simulink model "Explorer1632_dsPIC33EP512MU810_UART_Terminal_R2017b"  (R2017b)
settings: Solver=FixedStepDiscrete  StartTime=0.0  StopTime=inf  FixedStep=0.01  RelTol=1e-3  EnableMultiTasking=on
undefined symbols (not defined in the file): A0, D0, DiscIntNeverNeededParam, F4, F5, Max, ms, P100, P101, P16, P64, Pin, Resol, us
libraries: MCHP_Blockset x40, simulink x11
(part 1 of 2)
settings Model: ExtModeTrigDuration=1  Creator=M17129  LastModifiedBy=Lubin Kerhuel
settings OptimizationCC: DefaultParameterBehavior=Inlined  DefaultUnderspecifiedDataType=single  BooleansAsBitfields=on  PassReuseOutputArgsAs=Individual arguments
settings DebuggingCC: InheritedTsInSrcMsg=none  ParameterTunabilityLossMsg=error
settings HardwareCC: ProdBitPerInt=16  ProdBitPerPointer=32  ProdBitPerSizeT=16  ProdBitPerPtrDiffT=16  ProdLargestAtomicInteger=Integer  ProdLargestAtomicFloat=None  ProdWordSize=16  ProdHWDeviceType=Generic->Custom
settings ModelReferenceCC: ModelReferenceNumInstancesAllowed=Single
settings SFSimCC: MATLABDynamicMemAlloc=off
settings RTWCC: Description=Microchip Embedded Target PIC24 dsPIC30 dsPIC33 (real-time)  SystemTargetFile=MCHP_dsPIC_stf.tlc  TemplateMakefile=MCHP_dsPIC.tmf  GenerateReport=on  CustomInclude=./  CustomSource=code.c  IncludeHyperlinkInReport=on  LaunchReport=on  GenerateTraceInfo=on  GenerateTraceReport=on  GenerateTraceReportSl=on  GenerateTraceReportSf=on  GenerateTraceReportEml=on  GenerateWebview=on  GenerateCodeMetricsReport=on  GenerateCodeReplacementReport=on
settings CodeAppCC: ForceParamTrailComments=on  IgnoreCustomStorageClasses=off  MaxIdLength=255  OperatorAnnotations=on  SimulinkDataObjDesc=on  SFDataObjDesc=on  InsertBlockDesc=on
settings STFCustomTargetCC: TargetLibSuffix=_lib.a  MultiwordLength=256  IncludeMdlTerminateFcn=off  CombineOutputUpdateFcns=on  CombineSignalStateStructs=on  SuppressErrorStatus=on  ERTCustomFileBanners=on  SupportContinuousTime=off  RemoveResetFunc=on  MATLABClassNameForMDSCustomization=Simulink.SoftwareTarget.ERTCustomization  GRTInterface=off  SystemTargetFile=MCHP_dsPIC_stf.tlc
settings ERTTargetCC: TargetLibSuffix=_lib.a  ParMdlRefBuildCompliant=off  CompOptLevelCompliant=off  ConcurrentExecutionCompliant=off  IncludeMdlTerminateFcn=off  CombineSignalStateStructs=on  SuppressErrorStatus=on  SupportNonInlinedSFcns=on  ModelStepFunctionPrototypeControlCompliant=off  CPPClassGenCompliant=off  UseToolchainInfoCompliant=off  ExtModeStaticAllocSize=500  InlinedParameterPlacement=NonHierarchical  ERTSrcFileBannerTemplate=MCHP_dsPIC_code_template.cgt  ERTHdrFileBannerTemplate=MCHP_dsPIC_code_template.cgt  ERTDataSrcFileTemplate=MCHP_dsPIC_code_template.cgt  ERTDataHdrFileTemplate=MCHP_dsPIC_code_template.cgt  ERTCustomFileTemplate=MCHP_main.tlc  MemSecPackage=Simulink

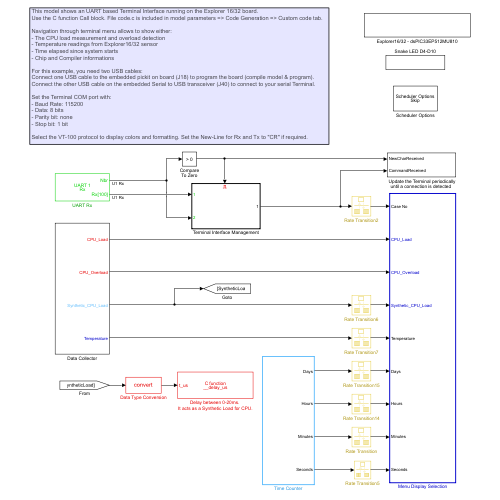
[thumbnail: Simulink's stored preview of the top-level diagram]
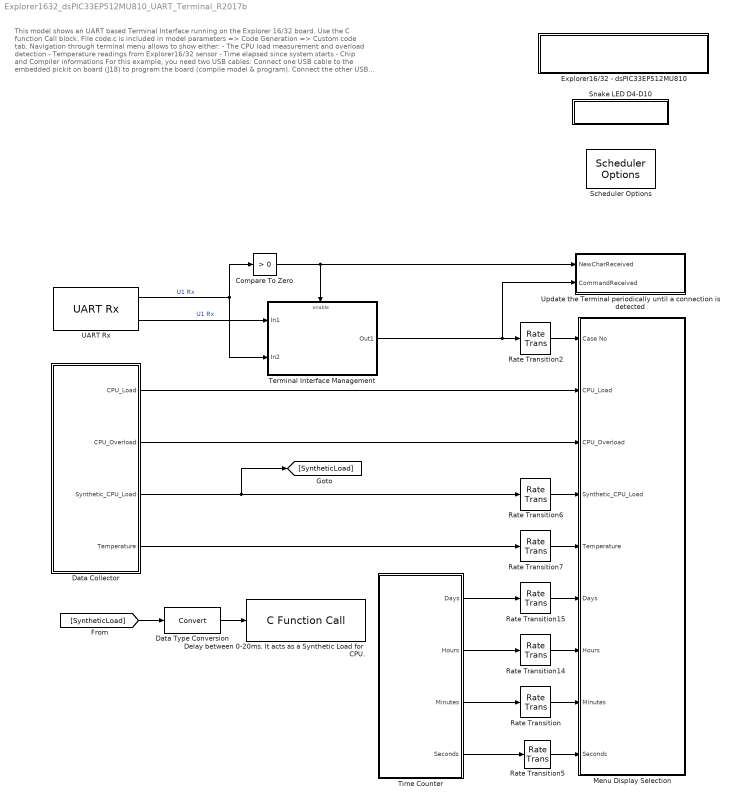
== system Explorer1632_dsPIC33EP512MU810_UART_Terminal_R2017b ==
  note: This model shows an UART based Terminal Interface running on the Explorer 16/32 board.
      | Use the C function Call block. File code.c is included in model parameters => Code Generation => Custom code tab.
      |
      | Navigation through terminal menu allows to show either:
      | - The CPU load measurement and overload detection
      | - Temperature readings from Explorer16/32 sensor
      | - Time elapsed since system starts
      | - Chip and Compiler informations
      |
      | For this example, you need two USB cables:
      | Connect one USB cable to the embedded pickit on board (J18) to program the board (compile model & program).
      | Connect the other USB cable on the embedded Serial to USB transceiver (J40) to connect to your serial Terminal.
      |
      | Set the Terminal COM port with:
      | - Baud Rate: 115200
      | - Data: 8 bits
      | - Parity bit: none
      | - Stop bit: 1 bit
      |
      | Select the VT-100 protocol to display colors and formatting. Set the New-Line for Rx and Tx to "CR" if required.
  " Update the Terminal periodically until a connection is detected " : Subsystem
  Compare To Zero : simulink/Logic and Bit Operations/Compare To Zero  relop=>  OutDataTypeStr=boolean
  Data Collector : Subsystem
  Data Type Conversion : DataTypeConversion
  Delay between 0-20ms. It acts as a Synthetic Load for CPU. : MCHP_Blockset/User Functions/C Function Call  ParseFilesChkbx=off  ListFunctions1=Custom Function  Function1=extern void __delay_us(unsigned long t_us);  AddHeaderDeclaration=off  Function1Type=when block is updated (default)  Fct1BlockIn=t_us  FctReturnBlockOut=off  DataCollected=0  ORDERING=None  SampleTime=-1  S_INPUT=0  S_INPUT_Size=0  S_OUTPUT=0  S_OUTPUT_Size=0  S_ListCustomDatatype=0  MCHP_CRC=957180  MCHP_MASTERLINK=Explorer1632_dsPIC33EP512MU810_UART_Terminal_R2017b/Explorer16//32 - dsPIC33EP512MU810/Microchip Master  PinDigitalInput=[]  PinDigitalOutput=[]  PinAnalogInput=[]
      settings: SourceProductName=MPLAB® Device Blocks for Simulink®
  Explorer16/32 - dsPIC33EP512MU810 : Subsystem
  Menu Display Selection : Subsystem  TreatAsAtomicUnit=on  SystemSampleTime=0.2
  Rate Transition{,2,5..7,14..15} (7 alike) : RateTransition  Deterministic=off  OutPortSampleTimeOpt=Inherit
  Scheduler Options : MCHP_Blockset/System Configuration/Scheduler Options  TaskOverloadBehaviour=Skip this task execution once  MCHP_MASTERLINK=UTester_33EP512MU810_CPUOverLoad/Microchip Master
      settings: SourceProductName=MPLAB® Device Blocks for Simulink®
  Snake LED D4-D10 : Subsystem
  Terminal Interface Management : Subsystem
  Time Counter : Subsystem  TreatAsAtomicUnit=on
  UART Rx : MCHP_Blockset/BUS UART/UART Rx  UART_REF=1  Flag_Out=on  Rx_Size_popup=User defined  Rx_Size=100  S_Rx_Size=100  Split=Read all received char  SplitChar=13  OutputDefault_popup=Add one trailing 0  OutputDefault=-2  ORDERING=None  SampleTime=0.01  MCHP_MASTERLINK=Explorer1632_dsPIC33EP512MU810_UART_Terminal_R2017b/Explorer16//32 - dsPIC33EP512MU810/Microchip Master  MCHP_COMPILED_INFO="CompiledSampleTime= [0.010000000000000000208   0 ];CompiledInportDataTypes=[    ];CompiledInportDataWidth=[];"
      settings: SourceProductName=MPLAB® Device Blocks for Simulink®
  wires:
  UART Rx/2 -> Terminal Interface Management/1(In1)  "U1 Rx"
  UART Rx/1 -> Terminal Interface Management/2(In2), Compare To Zero/1  "U1 Rx"
  Terminal Interface Management/1(Out1) -> Rate Transition2/1, " Update the Terminal periodically until a connection is detected "/2(CommandReceived)
  Data Collector/4(Temperature) -> Rate Transition7/1
  Time Counter/3(Minutes) -> Rate Transition/1
  Time Counter/1(Days) -> Rate Transition15/1
  Time Counter/2(Hours) -> Rate Transition14/1
  Time Counter/4(Seconds) -> Rate Transition5/1
  Rate Transition15/1 -> Menu Display Selection/6(Days)
  Rate Transition14/1 -> Menu Display Selection/7(Hours)
  Rate Transition/1 -> Menu Display Selection/8(Minutes)
  Rate Transition5/1 -> Menu Display Selection/9(Seconds)
  Compare To Zero/1 -> " Update the Terminal periodically until a connection is detected "/1(NewCharReceived), Terminal Interface Management/Enable
  Data Type Conversion/1 -> Delay between 0-20ms. It acts as a Synthetic Load for CPU./1
  Rate Transition2/1 -> Menu Display Selection/1(Case No)
  Data Collector/3(Synthetic_CPU_Load) -> [SyntheticLoad], Rate Transition6/1
  Data Collector/2(CPU_Overload) -> Menu Display Selection/3(CPU_Overload)
  Data Collector/1(CPU_Load) -> Menu Display Selection/2(CPU_Load)
  Rate Transition6/1 -> Menu Display Selection/4(Synthetic_CPU_Load)
  Rate Transition7/1 -> Menu Display Selection/5("Temperature ")
  [SyntheticLoad] -> Data Type Conversion/1

== system Explorer1632_dsPIC33EP512MU810_UART_Terminal_R2017b/ Update the Terminal periodically until a connection is detected  ==
  NewCharReceived : Inport
  CommandReceived : Inport  Port=2
  Logical Operator2 : Logic  Operator=OR  AllPortsSameDT=off  OutDataTypeStr=boolean
  Periodic update until a valid cmd is received : Subsystem
  Periodic update until first character is received : Subsystem
  Terminal Initialization : Subsystem  Priority=2
  wires:
  NewCharReceived/1 -> Periodic update until first character is received/1(NewCharReceived), Periodic update until a valid cmd is received/1(NewCharReceived)
  CommandReceived/1 -> Periodic update until a valid cmd is received/2(CommandReceived)
  Periodic update until a valid cmd is received/1(Update) -> Logical Operator2/2
  Logical Operator2/1 -> Terminal Initialization/Enable
  Periodic update until first character is received/1(Out1) -> Logical Operator2/1

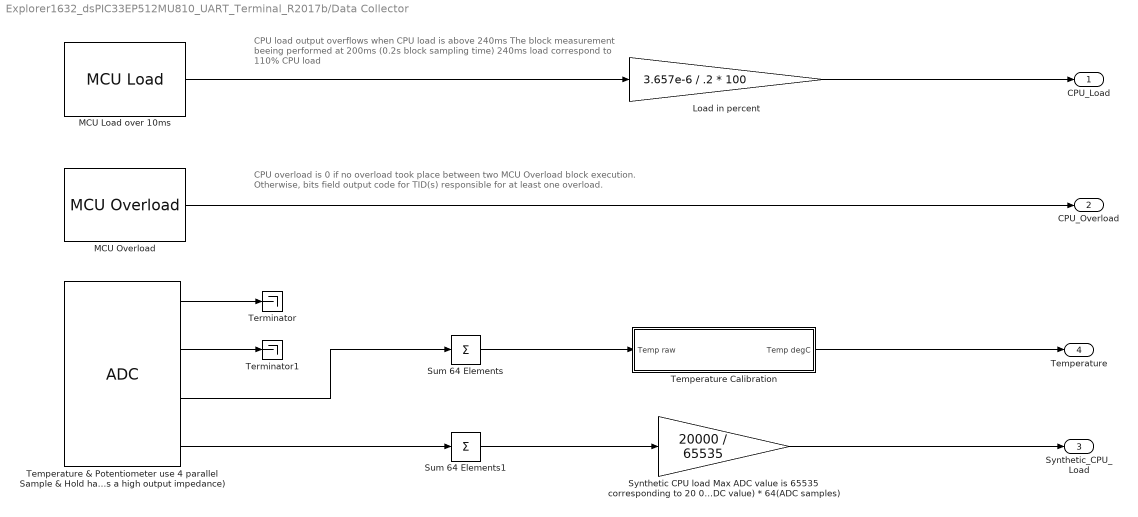
== system Explorer1632_dsPIC33EP512MU810_UART_Terminal_R2017b/Data Collector ==
  note: CPU overload is 0 if no overload took place between two MCU Overload block execution.
      | Otherwise, bits field output code for TID(s) responsible for at least one overload.
  note: CPU load output overflows when CPU load is above 240ms
      | The block measurement beeing performed at 200ms (0.2s block sampling time)
      | 240ms load correspond to 110% CPU load
  Load in percent : Gain  Gain=3.657e-6 / .2 * 100  ParamDataTypeStr=Inherit: Inherit from 'Gain'  OutMin=[0]  OutMax=[20]  OutDataTypeStr=single
  MCU Load over 10ms : MCHP_Blockset/Profiling/MCU Load  MCULoadPin=Dynamic Options  MCULoadPin_TXT=None  MCULoadMeasure=on  TIMER_Resolution=Dynamic Options  TIMER_Resolution_TXT="Resol: 3.657(us)  -  Max: 240(ms)"  MCHP_TIMER_REQUEST={MCU_Load}{MCU_Load}21:5:0:0:[]:16777216;  MCHP_TIMER_RESULT=[1 65535 ]  MCHP_MASTERLINK=Explorer1632_dsPIC33EP512MU810_UART_Terminal_R2017b/Explorer16//32 - dsPIC33EP512MU810/Microchip Master  MCHP_COMPILED_INFO="CompiledSampleTime= [0.2000000000000000111   0 ];CompiledInportDataTypes=[    ];CompiledInportDataWidth=[];"  Info="Timer 1:  Resol: 3.657142857(us)  -  Max: 239.675(ms)"  SampleTime=.2
      settings: SourceProductName=MPLAB® Device Blocks for Simulink®
  MCU Overload : MCHP_Blockset/Profiling/MCU Overload  MCUOverloadBlockOutput=on  MCUOverLoadPin=Dynamic Options  MCUOverLoadPin_TXT=None  MCHP_MASTERLINK=Explorer1632_dsPIC33EP512MU810_UART_Terminal_R2017b/Explorer16//32 - dsPIC33EP512MU810/Microchip Master  SampleTime=.2
      settings: SourceProductName=MPLAB® Device Blocks for Simulink®
  Sum 64 Elements : Sum  Inputs=+
  Sum 64 Elements1 : Sum  Inputs=+
  Synthetic CPU load Max ADC value is 65535 corresponding to 20 000us 65535(Max ADC Value) = 1024(10bit ADC value) * 64(ADC samples) : Gain  Gain=20000 / 65535  OutDataTypeStr=uint16
  Temperature & Potentiometer use 4 parallel Sample & Hold hardware (Temperature sensor has a high output impedance) : MCHP_Blockset/Analog IO/ADC  Priority=5  ADC_REF=1  Mode=10 bits (allows exact simultaneous sampling)  FORM=0000 dddd dddd dddd ==> Unsigned integer  ADC_R="< 10   kOhm"  nSAMPLECHANNELS=CH0 : CH1 : CH2 : CH3  nSAMPLECHANNELS_12bits=CH0 only  SIMULTANEOUS=Simultaneously on all Channels  ADxCSS=[0]  MUXA_CH0N=off  MUXA_CH123=Dynamic Options  MUXA_CH123_TXT=AN3 : AN4 : AN5  MUXB_CH0=AN1  MUXB_CH0N=on  MUXB_CH123=Dynamic Options  MUXB_CH123_TXT=AN0 : AN1 : AN2  SequenceRepeat=64  SequenceTiming=are stretcheded to fit exactly previous time step  SSRC_SSRCG=Dynamic Options  SSRC_SSRCG_TXT=6  Update_BlockOutput=After all trig and conversion sequence  Trig_TimeStep=with each update of the ADC block output  ADC_DMA_CHANNEL=use DMA Channel 0  SampleTime=0.01  Info=Total Time for Sample & Conversion : 0.0099968s including 5.8829e-05s (x 64) sample time. Difference with time step is : 3.2e-06s  MCHP_PORT={Analog Input 0}{AN0}15:2:B0;{Analog Input 3}{AN3}15:2:B3;{Analog Input 4}{AN4}15:2:B4;{Analog Input 5}{AN5}15:2:B5;  MCHP_MASTERLINK=Explorer1632_dsPIC33EP512MU810_UART_Terminal_R2017b/Explorer16//32 - dsPIC33EP512MU810/Microchip Master  ADC_TIMING=[0.0099968000000000001304]
      settings: SourceProductName=MPLAB® Device Blocks for Simulink®
  "Temperature Calibration " : Subsystem
  Terminator : Terminator
  Terminator1 : Terminator
  CPU_Load : Outport  VectorParamsAs1DForOutWhenUnconnected=off
  CPU_Overload : Outport  Port=2  VectorParamsAs1DForOutWhenUnconnected=off
  Synthetic_CPU_Load : Outport  Port=3  VectorParamsAs1DForOutWhenUnconnected=off
  Temperature : Outport  Port=4  VectorParamsAs1DForOutWhenUnconnected=off
  wires:
  Load in percent/1 -> CPU_Load/1
  MCU Load over 10ms/1 -> Load in percent/1
  Sum 64 Elements/1 -> "Temperature Calibration "/1(Temp raw)
  Temperature & Potentiometer use 4 parallel Sample & Hold hardware (Temperature sensor has a high output impedance)/3 -> Sum 64 Elements/1
  "Temperature Calibration "/1(Temp degC) -> Temperature/1
  Sum 64 Elements1/1 -> Synthetic CPU load Max ADC value is 65535 corresponding to 20 000us 65535(Max ADC Value) = 1024(10bit ADC value) * 64(ADC samples)/1
  Temperature & Potentiometer use 4 parallel Sample & Hold hardware (Temperature sensor has a high output impedance)/4 -> Sum 64 Elements1/1
  Synthetic CPU load Max ADC value is 65535 corresponding to 20 000us 65535(Max ADC Value) = 1024(10bit ADC value) * 64(ADC samples)/1 -> Synthetic_CPU_Load/1
  MCU Overload/1 -> CPU_Overload/1
  Temperature & Potentiometer use 4 parallel Sample & Hold hardware (Temperature sensor has a high output impedance)/1 -> Terminator/1
  Temperature & Potentiometer use 4 parallel Sample & Hold hardware (Temperature sensor has a high output impedance)/2 -> Terminator1/1

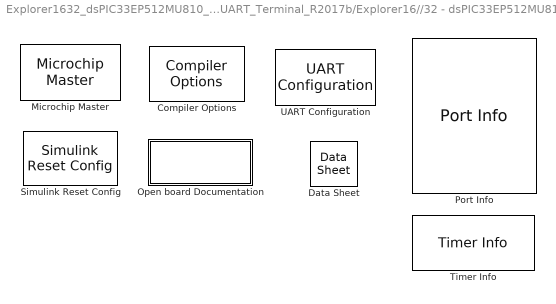
== system Explorer1632_dsPIC33EP512MU810_UART_Terminal_R2017b/Explorer16//32 - dsPIC33EP512MU810 ==
  Compiler Options : MCHP_Blockset/System Configuration/Compiler Options  Priority=1  LATEST_CMPLR=on  COMP_LIST=Dynamic Options  COMP_LIST_TXT=xc16 - v1.70  DFP_LIST=Dynamic Options  DFP_LIST_TXT=v 1.3.85  CMSIS_DSP=Dynamic Options  CMSIS_DSP_TXT=Dynamic Options  USE_64BIT_DOUBLE=off  MCHP_MULTITHREAD_COMPILATION=on  UseCustom_LinkerScript=off  MCHP_MASTERLINK=Explorer1632_dsPIC33EP512MU810_UART_Terminal_R2017b/Explorer16//32 - dsPIC33EP512MU810/Microchip Master  OPTIMIZATION_LEVEL=2  MPLAB_LINKLIB=default  MPLAB_LINKLIB1=default  CodeReplacement=Dynamic Options  CodeReplacement_TXT=None  OPTIMIZATION_FLTO=off  OPTIMIZATION_REORDER=off  UNROLL_LOOPS=off  PROCEDURAL_ABSTRACTION=off  MCODE=is less than 32768 (faster)  MCONST=in code memory  MDATA=Use only memory below address 8192 (faster)  MSCALAR=Use only memory below address 8192 (faster)  MLARGEARRAY=off  MAGGREGATE=on  HEAP_SIZE=0  OMF=elf  DEBUG_INFO=off  ProduceHexOutput=on  AssemblyListing=off  SaveTemps=off  NO_EDS_WARN=on  PRINT_STATISTICS=off
      settings: SourceProductName=MPLAB® Device Blocks for Simulink®
  Data Sheet : MCHP_Blockset/System Info/Data Sheet  DOC_Type=datasheet  DOC_MCHP_Id=33EP512MU810_datasheet  DOC_FilePath=C:\Users\M91449\AppData\Local\Temp\70616g.pdf  DOC_FileLastCheckTime="[2017              2             13             10              8         21.622]"  cpy_MCHP_Id=33EP512MU810  MCHP_MASTERLINK=Explorer1632_dsPIC33EP512MU810_UART_Terminal_R2017b/Explorer16//32 - dsPIC33EP512MU810/Microchip Master
      settings: AttributesFormatString=%<cpy_MCHP_Id>  SourceProductName=MPLAB® Device Blocks for Simulink®
  Microchip Master : MCHP_Blockset/System Configuration/Microchip Master  Priority=1  PICREF=33EP512MU810  TIMESTEP_REF="ADC  ( 0.01s + [-0.032%] ==> 0.0099968s )"  BUSYFLAG=A0 / Pin[17]  BUSYFLAG_TXT=A0 / Pin[17]  VDD_range=Dynamic Options  PWRTEN=Not used  BOREN=Disable  BODENV=2.7V  BORV=Not used  FPWRT=128ms  DSBOREN=Enable ZPBOR during Deep Sleep Mode  DSLPBOR=Not used  MCLRE=Enabled  SMCLR=MCLR pin generates a normal system Reset  PMDL1WAY=Allow only one reconfiguration  RSTPRI=Device will obtain reset instruction from Primary flash  TEMP=Not used  SOSCSRC=Not used  SOSCSEL=Not used  IOL1WAY=Allow only one reconfiguration  ALTVREF=Not used  DISUVREG=Not used  DSSWEN=Not used  LPCFG=Not used  RTCBAT=Not used  VBTBOR=Not used  WUTSEL=Not used  POWERSAVE=off  FNOSC=Primary Oscillator (XT; HS; EC)  FPR=ECIO w/ PLL 16x  FOSFPR=HS3 w/PLL 16x  FOS=Internal Fast RC  FRANGE=High Range  OSCILLATOR_SELECT=Crystal / Ceramic resonator  OSCILLATOR_SELECT_spd=Crystal / Ceramic resonator  QUARTZ=8e+06  QUARTZ_spd=8e+06  POSCGAIN=2x gain setting  POSCBOOST=Boost the kick start of the oscillator  SOSCGAIN=2x gain setting  SOSCBOOST=Boost the kick start of the oscillator  ACTIV_PLL=on  ACTIV_PLL_spd=on  MIPS_DESIRED=70e+06  MIPS_DESIRED_spd=70e+06  CPUDIV=Divide by 1  FPLLMUL=Not used  FPLLIDIV=8x Divider  POSCFREQ=Not used  POSCMD=XT Crystal Oscillator Mode  POSCMOD=Primary Oscillator Disabled  MIPS=70 * 1e6  ACLKCON=Optimized for PWM resolution & ADC conversion speed  ACLKCON_spd=Optimized for PWM resolution & ADC conversion speed  ACLKCON_Info=use FRC with auxilliary PLL, ADC Tad = 14.286(ns), PWM max resolution = 1.06(ns)  FPLLODIV=32x Divider  PLLKEN=Clock switch to PLL source will wait until the PLL lock signal is valid  FCKSM=Clock switching is enabled;Fail-safe Clock Monitor is disabled  FCKSMEN=Sw Disabled; Mon Disabled  IESO=Start up with FRC; then switch  DSWDTPS=1:2^36  FWDTEN=Disable  FWDTWINSZ=Window size is 25%  FWPSA=1:512  FWPSA0=1:128  FWPSB=1:16  WDT=Disable  WDTPOST=1:32768  WDTPRE=1:128  WDTPS=1:32768  WINDIS=Watchdog Timer in Non-Window mode  WWDTEN=Non-Window mode  DSWDTEN=Enable DSWDT during Deep Sleep Mode  DSWDTOSC=Select LPRC as DSWDT Reference clock  FPBDIV=Not used  FSOSCEN=Disable Secondary Oscillator  LPRCSEL=Not used  OSCIOFCN=Not used  OSCIOFNC=general purpose digital I/O pin  LVRCFG=Not used  PLL_96MHZ=Not used  PLL96MHZ=Not used  PLLDIV=Not used  WDTCLK=Not used  WDTCMX=Not used  WDTWIN=WDT Window is 25% of WDT period  XTCFG=24-32 MHz crystals  XTBST=Boost the kick-start  APL=Aux Flash Code protect is disabled  APLK=Aux Flash Write Protection and Code Protection is Disabled  AWRP=Auxiliary program memory is not write-protected  BSS=No Protection (other than BWRP)  BWP=Not used  BWRP=Boot Segment may be written  CP=Protection Disabled  EBS=No Boot EEPROM  ESS=No Segment Data EEPROM  GCP=General Segment Code protect is Disabled  GSS=General Segment Code protect is Disabled  GSS0=Not used  GSSK=General Segment Write Protection and Code Protection is Disabled  GWRP=General Segment may be written  PWP=Not used  RBS=No Boot RAM  RSS=No Secure RAM  SSS=No Secure Segment  SWRP=Secure segment may be written  WPCFG=Not used  WPDIS=Not used  WPEND=Not used  WPFP=Not used  ICESEL=Communicate on PGEC1/PGED1  ICS=Communicate on PGEC1 and PGED1  JTAGEN=Disable  COE=Not used  RES=Not used  DEBUG=Debugger is disabled  BACKBUG=Not used  BKBUG=Not used  ALTI2C=I2C mapped to SDA1/SCL1 pins  ALTI2C1=SDA1/SCK1 pins are selected as the I/O pins for I2C1  ALTI2C2=SDA2/SCK2 pins are selected as the I/O pins for I2C2  ALTI2C3=I2C3 mapped to SDA3/SCL3 pins  ALTQIO=QEA1; QEB1; INDX1 are selected as inputs to QEI1  ALTSS1=SS1A is selected as the I/O pin for SPI1  CMPPOL0=Hysteresis is applied to falling edge  CMPPOL1=Hysteresis is applied to falling edge  FCANIO=Not used  FETHIO=Default Ethernet I/O  FMIIEN=MII Enabled  FSRSSEL=Not used  FUSBIDIO=Controlled by the USB Module  FVBUSONIO=Not used  HPOL=Active High  HYST0=45 mV Hysteresis  HYST1=45 mV Hysteresis  I2C1SEL=Not used  LPOL=Active High  PWMPIN=Control with PORT/TRIS regs  RTCOSC=Not used  UPLLEN=USB PLL Disabled  UPLLIDIV=Not used  ATMOD8=Not used  ALTPMP=Not used  I2C2SEL=Not used  ALTADREF=Not used  ALTCVREF=Not used  PWMLOCK=PWM registers may be written without key sequence  INT_PRIORITY_DMA=0  MCHP_TIMER_RESULT=[ ]  MCHP_PORT={Busy Flag}{Busy}0:1:A0;  MCHP_PLLRegisters="[5    243  16385     -1     -1]"  MCHPVAR=MCHP.fcy.MIPS=70000000;MCHP.fcy.SYSCLK=70000000;MCHP.fcy.ADC=70000000;MCHP.fcy.Comparator=70000000;MCHP.fcy.I2C=70000000;MCHP.fcy.SPI=70000000;MCHP.fcy.UART=70000000;MCHP.fcy.Timers=70000000;MCHP.fcy.OC=70000000;MCHP.fcy.IC=70000000;MCHP.fcy.Ports=70000000;MCHP.fcy.QEI=70000000;MCHP.PowerSave=0;MCHP.TimeStepFactor=0.99968;MCHP.TimeStep_Timer=-1;MCHP.NTIMERS=9;MCHP.id.name='33EP512MU810';MCHP.id.N=reshape([33 512 810],1,3);MCHP.id.L=reshape({ 'EP','MU',''},1,3);MCHP.id.Arch=3;MCHP.periph.PPS.reg_RPINRx=reshape([-1 1 1 1 1 -1 1 1 1 1 1 1 1 1 1 1 1 1 1 1 1 1 -1 -1 1 1 1 1 1 1 1 1 1 1 1 1 1 1 1 1 1 1 1 -1 -1 -1 1 -1 -1 -1 -1 -1 1 1 1 1 1 1 1 1 1 -1 1 1 1 -1 1 1 1 1 1 1 1 1 -1 1 1 1 1 1 1 1 1 -1 1 1 1],1,87);MCHP.PPS.dsPIC.RP=reshape([-1 -1 -1 -1 -1 -1 -1 -1 -1 -1 -1 -1 -1 -1 -1 -1 -1 -1 -1 -1 -1 -1 -1 -1 -1 -1 -1 -1 -1 -1 -1 -1 -1 -1 -1 -1 -1 -1 -1 -1 -1 -1 -1 -1 -1 -1 -1 -1 -1 -1 -1 -1 -1 -1 -1 -1 -1 -1 -1 -1 -1 -1 -1 -1 48 49 50 51 52 53 54 55 -1 -1 -1 -1 -1 -1 -1 63 64 -1 66 -1 68 69 -1 71 -1 -1 -1 -1 -1 -1 -1 -1 80 81 82 83 84 85 -1 -1 88 -1 -1 -1 92 93 -1 -1 96 97 -1 -1 -1 -1 102 -1 104 -1 -1 -1 -1 109 110 111],1,128);MCHP.PPS.dsPIC.RPI=reshape([-1 -1 -1 -1 -1 -1 -1 -1 -1 -1 -1 -1 -1 -1 -1 -1 0 1 2 3 4 5 6 7 -1 -1 -1 -1 -1 -1 14 15 16 17 18 19 20 21 22 23 24 25 26 27 28 29 30 31 -1 33 34 35 36 -1 -1 -1 -1 -1 -1 -1 44 45 46 -1 -1 -1 -1 -1 -1 -1 -1 -1 56 57 58 59 60 61 62 -1 -1 65 -1 67 -1 -1 70 -1 72 73 -1 -1 -1 -1 -1 -1 -1 -1 -1 -1 -1 -1 -1 -1 -1 -1 -1 -1 -1 -1 -1 -1 -1 -1 -1 -1 -1 -1 -1 103 -1 105 -1 -1 108],1,125);MCHP.PPS.dsPIC.RPINR_list=reshape({ '1','INT1','INT2','INT3','INT4','T1CK','T2CK','T3CK','T4CK','T5CK','T6CK','T7CK','T8CK','T9CK','IC1','IC2','IC3','IC4','IC5','IC6','IC7','IC8','OCFA','OCFB','FLT1','FLT2','FLT3','FLT4','QEIA1','QEIB1','QEINDX1','QEIHOM1','QEIA2','QEIB2','QEINDX2','QEIHOM2','U1RX','U1CTS','U2RX','U2CTS','SDI1','SCK1_in','SS1_in','44','SDI2','SCK2_in','SS2_in','48','CSDIR','CSCK','COFS','52','C1RX','C2RX','U3RX','U3CTS','U4RX','U4CTS','SDI3','SCK3_in','SS3_in','62','SDI4','SCK4_in','SS4_in','66','IC9','IC10','IC11','IC12','IC13','IC14','IC15','IC16','OCFC','SYNCI1','SYNCI2','DTCMP1','DTCMP2','DTCMP3','DTCMP4','DTCMP5','DTCMP6','DTCMP7','FLT5','FLT6','FLT7','FLT8','89','SENT1','SENT2','92'},1,92);MCHP.PPS.dsPIC.RPOR_list=reshape({ '1','U1TX','U1RTS','U2TX','U2RTS','SDO1','SCK1_out','SS1_out','SDO2','SCK2_out','SS2_out','CSDO','CSCK','COFS','C1TX','C2TX','OC1','OC2','OC3','OC4','OC5','OC6','OC7','OC8','C1OUT','C2OUT','C3OUT','U3TX','U3RTS','U4TX','U4RTS','SDO3','SCK3_out','SS3_out','SDO4','SCK4_out','SS4_out','OC9','OC10','OC11','OC12','OC13','OC14','OC15','OC16','SYNCO1','SYNCO2','QEI1CCMP','QEI2CCMP','REFCLK','C4OUT','C5OUT','52','53','54','55','56','SENT1','SENT2'},1,59);MCHP.PPS.map_RPnR_RPORx=reshape([64 65 66 67 68 69 70 71 79 80 82 84 85 87 96 97 98 99 100 101 -1 -1 104 108 109 112 113 118 120 125 126 127],1,32);MCHP.Rx=reshape([17 25 -1 72 93 87 90 -1 -1 -1 -1 38 24 6 76 94 88 89 -1 -1 -1 -1 58 23 7 77 98 52 57 -1 -1 -1 -1 59 22 8 78 99 51 56 -1 -1 -1 -1 60 21 9 81 100 49 -1 -1 -1 -1 -1 61 20 -1 82 3 50 -1 -1 -1 -1 -1 91 26 -1 83 4 -1 10 -1 -1 -1 -1 92 27 -1 84 5 -1 11 -1 -1 -1 -1 -1 32 -1 68 18 53 12 -1 -1 -1 -1 28 33 -1 69 19 -1 14 -1 -1 -1 -1 29 34 -1 70 -1 -1 -1 -1 -1 -1 -1 -1 35 -1 71 -1 -1 -1 -1 -1 -1 -1 -1 41 63 79 -1 40 96 -1 -1 -1 -1 -1 42 73 80 -1 39 97 -1 -1 -1 -1 66 43 74 47 -1 -1 95 -1 -1 -1 -1 67 44 64 48 -1 -1 1 -1 -1 -1 -1],11,16);MCHP.ADC.ANtype=reshape([3 1],1,2);MCHP.ADC.ADCONx=reshape([47103 59391 40959 263 0 0],1,6);MCHP.ADC.ADCHS_0=reshape([40863 1799],1,2);MCHP.ADC.Flags=reshape([1 0],1,2);MCHP.ADC.Buffer=reshape([16 16],1,2);MCHP.ADC.port=reshape([16 17 18 19 20 21 22 23 24 25 26 27 28 29 30 31 33 34 35 36 72 73 6 7 64 65 66 67 68 69 70 71 -1 -1 -1 -1 -1 -1 -1 -1 -1 -1 -1 -1 -1 -1 -1 -1 -1 -1 -1 -1 -1 -1 -1 -1 -1],1,57);MCHP.ADC.port_ALT=reshape([-1 -1 -1 -1],1,4);MCHP.ADC.port_VrefP=10;MCHP.ADC.port_VrefM=9;MCHP.ADC.port_AVdd=-1;MCHP.ADC.port_AVss=-1;MCHP.ADC.ADCDATA=reshape([0 0 0 0 0 0 0 0 0 0 0 0 0 0 0 0 0 0 0 0 0 0 0 0 0 0 0 0 0 0 0 0 0 0 0 0 0 0 0 0 0 0 0 0 0 0 0 0 0 0 0 0 0 0 0 0 0],1,57);MCHP.ADC.HS_SAR.TRGSRC=reshape([0 0 0 0 0 0 0 0 0 0 0 0 0 0 0 0 0 0 0 0 0 0 0 0 0 0],1,26);MCHP.ADC.HS_SAR.nFilters=0;MCHP.ADC.HS_SAR.nDedicatedCore=0;MCHP.ADC.HS_SAR.CALIBRATION=0;MCHP.ADC.HS_SAR.ADCON1L=-1;MCHP.ADC.HS_SAR.ADC_Class3_idxStart=32;MCHP.memory.RAM=53248;MCHP.memory.RAM_XBegin=4096;MCHP.memory.RAM_YBegin=36864;MCHP.memory.RAM_dma=reshape([53248 57344],1,2);MCHP.memory.FLASH_ECC=0;MCHP.DMA.Num=15;MCHP.DMA.CNTmax=16383;MCHP.QEI.QEICONx=reshape([49023 49023 -1 -1 -1 -1],1,6);MCHP.QEI.QEItype=2;MCHP.QEI.Port_QEI_INDX=reshape([-1 -1],1,2);MCHP.QEI.Port_QEI_QEA=reshape([-1 -1],1,2);MCHP.QEI.Port_QEI_QEB=reshape([-1 -1],1,2);MCHP.QEI.Port_QEI_UPDN=reshape([-1 -1],1,2);MCHP.INT.Port=reshape([48 32767 32767 32767 32767],1,5);MCHP.PWM_HS.Flags=reshape([6 2 1],1,3);MCHP.PWM.port_FLT=reshape([-1 -1 -1 -1 -1 -1 -1 -1 -1 -1 -1 -1 -1 -1 -1 -1 -1 -1 -1 -1 -1 -1 -1 -1 -1 -1 -1 -1 -1 -1 -1 -1 -1],1,33);MCHP.PWM.PWMRef=-1;MCHP.PWM.Flag=0;MCHP.PWM.Port_PWM_l=reshape([64 -1 66 -1 68 -1 70 -1 33 -1 35 -1 -1 -1 -1 -1 -1 -1 -1 -1 -1 -1 -1 -1],2,12);MCHP.PWM.Port_PWM_h=reshape([65 -1 67 -1 69 -1 71 -1 34 -1 36 -1 -1 -1 -1 -1 -1 -1 -1 -1 -1 -1 -1 -1],2,12);MCHP.PWM_HS_FEP.nEVTOUT=-1;MCHP.IC.Port=reshape([32767 32767 32767 32767 32767 32767 32767 32767 32767 32767 32767 32767 32767 32767 32767 32767],1,16);MCHP.IC.type=1;MCHP.OC.Port=reshape([32767 32767 32767 32767 32767 32767 32767 32767 32767 32767 32767 32767 32767 32767 32767 32767],1,16);MCHP.OC.type=1;MCHP.CN.Port=reshape([-1 -1 -1 -1 -1 -1 -1 -1 -1 -1 -1 -1 -1 -1 -1 -1 -1 -1 -1 -1 -1 -1 -1 -1 -1 -1 -1 -1 -1 -1 -1 -1 -1 -1 -1 -1 -1 -1 -1 -1 -1 -1 -1 -1 -1 -1 -1 -1 -1 -1 -1 -1 -1 -1 -1 -1 -1 -1 -1 -1 -1 -1 -1 -1 -1 -1 -1 -1 -1 -1 -1 -1 -1 -1 -1 -1 -1 -1 -1 -1 -1 -1 -1 -1 -1],1,85);MCHP.CN.PullUp=reshape([50943 65535 61470 65535 1023 12607 62403 0 0 0 0],1,11);MCHP.CN.type=1;MCHP.CN.Flag_PullDown=1;MCHP.SPI.Refs=reshape([1 2 3 4 0 0],1,6);MCHP.SPI.SPIxCON1=8191;MCHP.SPI.SPIxCON2=57347;MCHP.SPI.Port_SDI=reshape([-1 103 -1 -1 -1 -1],1,6);MCHP.SPI.Port_SDO=reshape([-1 104 -1 -1 -1 -1],1,6);MCHP.SPI.Port_SCK=reshape([-1 102 -1 -1 -1 -1],1,6);MCHP.SPI.Port_SS=reshape([-1 -1 -1 -1 -1 -1],1,6);MCHP.I2C.Refs=reshape([1 2 0 0 0],1,5);MCHP.I2C.I2CxCON=49151;MCHP.I2C.NewRegName=1;MCHP.I2C.Port_SDA=reshape([-1 84 -1 -1 -1],1,5);MCHP.I2C.Port_SCL=reshape([-1 85 -1 -1 -1],1,5);MCHP.I2C.Port_ASDA=reshape([57 3 -1 -1 -1],1,5);MCHP.I2C.Port_ASCL=reshape([58 2 -1 -1 -1],1,5);MCHP.I2C.Fuse_Port_SCL_SDA=reshape([17 1 18 1 -1 -1 -1 -1 -1 -1],2,5);MCHP.I2C.Fuse_Port_ASCL_ASDA=reshape([17 2 18 2 -1 -1 -1 -1 -1 -1],2,5);MCHP.SCCP.nSCCP=0;MCHP.SCCP.MCCP=reshape([0 0 0 0 0 0 0 0 0],1,9);MCHP.PGA.Port_PGA1P=reshape([-1 -1 -1 -1],1,4);MCHP.PGA.Port_PGA1N=reshape([-1 -1 -1 -1],1,4);MCHP.PGA.Port_PGA2P=reshape([-1 -1 -1 -1],1,4);MCHP.PGA.Port_PGA2N=reshape([-1 -1 -1 -1],1,4);MCHP.PGA.Num=0;MCHP.HS_AnalogComparator.Port_CMP1=reshape([-1 -1 -1 -1],1,4);MCHP.HS_AnalogComparator.Port_CMP2=reshape([-1 -1 -1 -1],1,4);MCHP.HS_AnalogComparator.Port_CMP3=reshape([-1 -1 -1 -1],1,4);MCHP.HS_AnalogComparator.Port_CMP4=reshape([-1 -1 -1 -1],1,4);MCHP.HS_AnalogComparator.PORT_EXTREFx=reshape([-1 -1],1,2);MCHP.HS_AnalogComparator.Port_DACOUTx=reshape([-1 -1],1,2);MCHP.HS_AnalogComparator.Num=0;MCHP.Comp.Port_CVrefin=-1;MCHP.Comp.Port_CVref=26;MCHP.Comp.Port_CVref1O=-1;MCHP.Comp.Port_CVref2O=-1;MCHP.Comp.Port_CxOUT=reshape([32767 32767 32767 -1 -1],1,5);MCHP.Comp.Port_OAxOUT=reshape([-1 -1 -1 -1 -1],1,5);MCHP.Comp.Port_CxINP=reshape([21 19 55 -1 -1],1,5);MCHP.Comp.Port_CxINM=reshape([103 20 102 -1 105 18 104 -1 46 54 45 -1 -1 -1 -1 -1 -1 -1 -1 -1],4,5);MCHP.Comp.Port_OAxINP=reshape([-1 -1 -1 -1 -1],1,5);MCHP.Comp.Port_OAxINM=reshape([-1 -1 -1 -1 -1],1,5);MCHP.Comp.nComp=reshape([3 0 0],1,3);MCHP.Comp.OpAmp=0;MCHP.Comp.CVRCON=reshape([2047 0],1,2);MCHP.Comp.CMCON=0;MCHP.CDAC.Port_DACx=reshape([-1 -1 -1],1,3);MCHP.CDAC.nCDAC=0;MCHP.UART.port_Rx=reshape([32767 32767 32767 32767 -1 -1],1,6);MCHP.UART.port_Tx=reshape([32767 32767 32767 32767 -1 -1],1,6);MCHP.UART.port_ARx=reshape([-1 -1],1,2);MCHP.UART.port_ATx=reshape([-1 -1],1,2);MCHP.UART.port_RTS=reshape([32767 32767 32767 32767 -1 -1],1,6);MCHP.UART.port_CTS=reshape([32767 32767 32767 32767 -1 -1],1,6);MCHP.UART.reg_UxMODE=reshape([48127 48127 48127 48127 -1 -1],1,6);MCHP.UART.reg_UxSTA=reshape([61439 61439 61439 61439 -1 -1],1,6);MCHP.modsrc.DOS_02551_cpu_16bit_v7=0;MCHP.modsrc.DOS_01520_wdt_dmt_upb_v1_16bit=0;MCHP.modsrc.DOS_02359a_sent_j2716_upb_v1=0;MCHP.modsrc.DOS_02672_math_progcrc_upb_v1_16bit=0;MCHP.modsrc.DOS_01577_cla_clc_upb_v1=0;MCHP.modsrc.DOS_02915_ecc_v2=0;MCHP.modsrc.DOS_02673_tmr_classa_upb_v1_16bit=0;MCHP.modsrc.DOS_01494_qei_32b_upb_v1_16bit=0;MCHP.modsrc.DOS_02552_msi_upb_v1_Master=0;MCHP.modsrc.DOS_01441_i2c_upb_v1_16bit_TLAH=0;MCHP.modsrc.DOS_03076_uart_protocol_upb_v1_16bit=0;MCHP.modsrc.DOS_01482=0;MCHP.modsrc.DOS_01483_pwm_16bit=0;MCHP.modsrc.DOS_02497_WACV=0;MCHP.modsrc.DOS_02316_nvm_ctrl_v1_16bit=0;MCHP.modsrc.DOS_02653_afe_current_bias_ctrl_upb_v1_16bit=0;MCHP.modsrc.DOS_01459_ptg_pc_upb_v1_16bit=0;MCHP.modsrc.DOS_01512_ccp_mccp_upb_v1_16bit=0;MCHP.modsrc.DOS_02519_dma_sfr_16bit_v2=0;MCHP.modsrc.DOS_02508c11=0;MCHP.modsrc.DOS_02475_dac_pdm_nbit_upb_v1_16bit=0;MCHP.modsrc.DOS_02467_gpio_upb_v1_16bit=0;MCHP.modsrc.DOS_00805_rst_integration_v4=0;MCHP.modsrc.DOS_02659_clk_sib_v12=0;MCHP.modsrc.DOS_02674_wdt_upb_v1_16bit=0;MCHP.modsrc.DOS_01407=0;MCHP.modsrc.DOS_02552_msi_upb_v1_Slave=0;MCHP.modsrc.DOS_02593_amp_pga_ctrl_pb_v2_16bit=0;MCHP.modsrc.DOS_03247_CAN_FD_UPB_V2_16_bit=0;MCHP.modsrc.DOS_01461_afe_ctmu_con_upb_v1_16bit=0;MCHP.modsrc.DOS_02497_WACA=0;MCHP.modsrc.DOS_02478_uart_irda_upb_v1_16bit=0;MCHP.modsrc.DOS_00929=1;MCHP.modsrc.DOS_01198=1;MCHP.modsrc.DOS_03029_WACH=0;MCHP.modsrc.DOS_02949_WACG=0;MCHP.modsrc.DOS_03349_amp_pad_opamp_ctrl_upb_v1=0;MCHP.modsrc.DOS_02237_osc_dco_ctrl_upb_v1_16bit=0;MCHP.modsrc.DOS_02472_ppi_pmp16_upb_v1_16bit=0;MCHP.modsrc.DOS_03994_WAC07=0;MCHP.modsrc.DOS_03662_WACU=0;MCHP.modsrc.DOS_00794=1;MCHP.modsrc.DOS_00931=1;MCHP.modsrc.DOS_00932=1;MCHP.modsrc.DOS_00942=1;MCHP.modsrc.DOS_00938=1;MCHP.modsrc.DOS_00996=1;MCHP.modsrc.DOS_00997=1;MCHP.modsrc.DOS_00998=1;MCHP.modsrc.DOS_00209=1;MCHP.modsrc.DOS_01555_adc=0;MCHP.modsrc.DOS_01293=0;MCHP.modsrc.DOS_00828=1;MCHP.modsrc.DOS_01116=1;MCHP.modsrc.DOS_01017_RPORx=1;MCHP.modsrc.DOS_01017_RPINRx=1;MCHP.modsrc.DOS_01555_nvm_tsmc18_v2_16bit=0;MCHP.modsrc.DOS_00804=1;MCHP.modsrc.DOS_00826=1;MCHP.modsrc.DOS_01555_TLAK_PMDx=0;MCHP.modsrc.DOS_01555_TLAK_INT_=0;MCHP.modsrc.DOS_00933=1;MCHP.modsrc.DOS_01555=0;MCHP.modsrc.DOS_01555_ptg=0;MCHP.modsrc.DOS_00958=1;MCHP.modsrc.DOS_01117_PORTx=1;MCHP.modsrc.DOS_00999=1;MCHP.modsrc.DOS_01041=1;MCHP.modsrc.DOS_00892=1;MCHP.modsrc.DOS_01287_TLAC_PMDx=0;MCHP.modsrc.DOS_01287_TLAC_INT_=0;MCHP.modsrc.DOS_01424=0;MCHP.modsrc.DOS_01332=0;MCHP.modsrc.DOS_01468_PMBA_current_source=0;MCHP.modsrc.DOS_02291_PGA=0;MCHP.modsrc.DOS_01467_Comparator=0;MCHP.modsrc.DOS_01498_TLAY=0;MCHP.modsrc.DOS_00993_PLL_120MHz=0;MCHP.modsrc.DOS_01332_ptg_pc_v1=0;MCHP.modsrc.DOS_00958_pwm_TLAY=0;MCHP.modsrc.TLAY_IOPorts=0;MCHP.modsrc.DOS_00929q=0;MCHP.modsrc.DOS_02415_spi_v5=0;MCHP.modsrc.DOS_RPINRx_16bit_2=0;MCHP.modsrc.DOS_01497_TLAH_PMDx=0;MCHP.modsrc.DOS_02550_TLAL_INT=0;MCHP.modsrc.DOS_00958_pwm_TLAH=0;MCHP.modsrc.DOS_01287_TLAH_INT_=0;MCHP.modsrc.DOS_01113=1;MCHP.modsrc.DOS_01017_PMDx=1;MCHP.modsrc.DOS_00927=1;MCHP.modsrc.DOS_01080=1;MCHP.modsrc.DOS_00794_cpu_16bit_v3=0;MCHP.modsrc.DOS_02192_TLCD_PMDx=0;MCHP.modsrc.DOS_02192_TLCD_INT_=0;MCHP.modsrc.DOS_02192_cmp=0;MCHP.modsrc.DOS_00958_pwm_TLCD=0;MCHP.modsrc.DOS_02192_PORTx_TLCD=0;MCHP.modsrc.DOS_00936=0;MCHP.modsrc.DOS_00995=0;MCHP.modsrc.DOS_00546=0;MCHP.modsrc.DOS_00474=0;MCHP.modsrc.DOS_02481_WACK_MC_Config=0;MCHP.modsrc.DOS_03088_pfm_cache_ocp_v2_WACK=0;MCHP.modsrc.DOS_02819_pfm_ctrl_32bit_upb_v2=0;MCHP.modsrc.DOS_02674_wdt_upb_v1_32bit=0;MCHP.modsrc.DOS_01520_wdt_dmt_upb_v1=0;MCHP.modsrc.DOS_02869_icd_jtag_bvci_upb_v2=0;MCHP.modsrc.DOS_02823_WACJ_clk_cru_upb_v2=0;MCHP.modsrc.DOS_02823_WACN_clk_cru_upb_v2=0;MCHP.modsrc.DOS_01423_RPINRx=0;MCHP.modsrc.DOS_02481_RPORx=0;MCHP.modsrc.DOS_02511_pwr_sib_upb_v1_32bit=0;MCHP.modsrc.DOS_02907_WACN_GP_int_evic_v3=0;MCHP.modsrc.DOS_01500_dma_bvci_v2=0;MCHP.modsrc.DOS_02141_tmr_classa_pb_v2=0;MCHP.modsrc.DOS_02815_tmr_classb_upb_v1=0;MCHP.modsrc.DOS_00740_icap_pb_v1=0;MCHP.modsrc.DOS_00749_ocmp_pb_v1=0;MCHP.modsrc.DOS_01441_i2c_upb_v1_32bit=0;MCHP.modsrc.DOS_01329_spi_pb_v2=0;MCHP.modsrc.DOS_02478_uart_irda_upb_v1_32bit=0;MCHP.modsrc.DOS_03554_cmp_control_upb_v2_32bit=0;MCHP.modsrc.DOS_01445_dac_nbit__control_upb_v1_32bit=0;MCHP.modsrc.DOS_01461_afe_ctmu_con_upb_v1=0;MCHP.modsrc.DOS_01577_cla_clc_upb_v1_32bit=0;MCHP.modsrc.DOS_02467_gpio_ports_upb_v1=0;MCHP.modsrc.DOS_02508_adc_sar_ctrl_upb_v1_PIC32MK=0;MCHP.modsrc.DOS_01261_tmr_rtcc_pb_v2=0;MCHP.modsrc.DOS_01475_lpwr_deep_sleep_ctrl_v2=0;MCHP.modsrc.DOS_EIP_00136_ssx_v1=0;MCHP.modsrc.DOS_02907_WACN_MC_int_evic_v3=0;MCHP.modsrc.DOS_01477_pwm_mc_upb_v1=0;MCHP.modsrc.DOS_01494_qei_32b_upb_v1=0;MCHP.modsrc.DOS_03247_can_fd_upb_v2_pic32mk=0;MCHP.modsrc.DOS_02907_WACK_MC_int_evic_v3=0;MCHP.modsrc.DOS_02514_dfm_strl_sst_upb_v1=0;MCHP.modsrc.DOS_02472_ppi_pmp16_upb_v1=0;MCHP.modsrc.DOS_02813a_usb_otgcore_pb_v3=0;MCHP.modsrc.DOS_02481_WACJ_MC_Config=0;MCHP.modsrc.DOS_02569_pfm_cache_ocp_v1=0;MCHP.modsrc.DOS_02481_WACJ_MC_int_evic_v3=0;MCHP.modsrc.DOS_01459_ptg_pc_upb_v1_SIC=0;MCHP.modsrc.DOS_01427_cmp_control_upb_v1_32bit=0;MCHP.modsrc.DOS_01152_can_bvci_v1=0;MCHP.modsrc.DOS_02787_WACD_Config=0;MCHP.modsrc.DOS_00800_dac_4bit_ctrl_pb_v1=0;MCHP.modsrc.DOS_01539_icd_jtag_pb_v2=0;MCHP.modsrc.DOS_02823_clk_cru_upb_v2=0;MCHP.modsrc.DOS_01423_RPORx=0;MCHP.modsrc.DOS_02907_WACD_int_evic_v3=0;MCHP.modsrc.DOS_00734_uart_irda_pb_v1=0;MCHP.modsrc.DOS_00687_tmr_classa_pb_v1=0;MCHP.modsrc.DOS_00745_tmr_classb_pb_v1=0;MCHP.modsrc.DOS_02508_adc_sar_ctrl_upb_v1=0;MCHP.modsrc.DOS_00866_cmp_control_pb_v2=0;MCHP.modsrc.DOS_01114_eth_bvci_v1=0;MCHP.modsrc.DOS_02831_usb_clk_rst_v2=0;MCHP.modsrc.DOS_01643_pfm_cache_ahb_v2=0;MCHP.modsrc.DOS_EIP_00206r5_sqi_v2=0;MCHP.modsrc.DOS_EIP_00124_usb_hs_otgcore_v1=0;MCHP.modsrc.DOS_EIP_00218_math_rng_ahbs_v2=0;MCHP.modsrc.DOS_EIP_00109_ebi_v1=0;MCHP.modsrc.DOS_EIP_00158_crypto_v1=0;MCHP.PortBase=16;MCHP.PortPrefixe='P';MCHP.clock.PBxDIV=-1;  MCHP_CRC=15032026  BTMODE=Not used  RES1=Not used  PLLSS=Not used  RES2=Not used  ALTCMPI=Not used  BOREN1=Not used  ALTRB6=Not used  RETCFG=Not used  DFMCY=Not used  BSS2=No Boot Segment  BSEN=No Boot Segment  CWRP=Configuration Segment may be written  CSS=No Protection (other than CWRP)  AIVTDIS=Disabled AIVT  BSLIM=Not used  WDTEN=Disable  BTSWP=BOOTSWP instruction is disabled  DBCC=No Cross Connection between DAC outputs  CTXT1=Not Assigned  CTXT2=Not Assigned  SEQNUM=Not used  nSEQNUM=Not used  BOREN0=Enabled  DMTIVT=Not used  DMTCNT=2^31 (2147483648)  DMTEN=Dead Man Timer is Disabled and can be enabled by software  ON=Not used  USERID=Not used  RESERVED1=Not used  PGL1WAY=Allow only one reconfiguration  FPLLRNG=34-68 MHz Input  FPLLICLK=FRC is input to the System PLL  FPLLMULT=PLL Multiply by 128  UPLLFSEL=USB PLL input is 24 MHz  DMTINTV=Window/Interval value is 127/128 counter value  WDTSPGM=WDT stops during Flash programming  FDMTEN=Deadman Timer is disabled  TRCEN=Trace features in the CPU are enabled  BOOTISA=Boot code and Exception code is MIPS32  FECCCON=ECC and Dynamic ECC are disabled (ECCCON bits are writable)  EXTDDRSIZE=Not used  FSLEEP=Flash is powered down when the device is in Sleep mode  DBGPER=Allow CPU access to all permission regions  EJTAGBEN=Normal EJTAG functionality  TSEQ=Not used  CSEQ=Not used  RWDTPS=1:1048576  RCLKSEL=Always use LPRC  SWDTPS=1:1048576  DMTIVTL=Not used  DMTIVTH=Not used  DMTCNTL=Not used  DMTCNTH=Not used  DMTDIS=Dead Man Timer is Disabled and can be enabled by software  SMBEN=SMBus input threshold is enabled  SPI2PIN=SPI2 uses I/O remap (PPS) pins  CTXT3=Not Assigned  CTXT4=Not Assigned  MBXM0=Mailbox register configured for Master data read (Slave to Master data transfer)  MBXM1=Mailbox register configured for Master data read (Slave to Master data transfer)  MBXM2=Mailbox register configured for Master data read (Slave to Master data transfer)  MBXM3=Mailbox register configured for Master data read (Slave to Master data transfer)  MBXM4=Mailbox register configured for Master data read (Slave to Master data transfer)  MBXM5=Mailbox register configured for Master data read (Slave to Master data transfer)  MBXM6=Mailbox register configured for Master data read (Slave to Master data transfer)  MBXM7=Mailbox register configured for Master data read (Slave to Master data transfer)  MBXM8=Mailbox register configured for Master data read (Slave to Master data transfer)  MBXM9=Mailbox register configured for Master data read (Slave to Master data transfer)  MBXM10=Mailbox register configured for Master data read (Slave to Master data transfer)  MBXM11=Mailbox register configured for Master data read (Slave to Master data transfer)  MBXM12=Mailbox register configured for Master data read (Slave to Master data transfer)  MBXM13=Mailbox register configured for Master data read (Slave to Master data transfer)  MBXM14=Mailbox register configured for Master data read (Slave to Master data transfer)  MBXM15=Mailbox register configured for Master data read (Slave to Master data transfer)  MBXHSA=MSIxMBXD15 assigned to mailbox handshake protocol block A  MBXHSB=MSIxMBXD15 assigned to mailbox handshake protocol block B  MBXHSC=MSIxMBXD15 assigned to mailbox handshake protocol block C  MBXHSD=MSIxMBXD15 assigned to mailbox handshake protocol block D  MBXHSE=MSIxMBXD15 assigned to mailbox handshake protocol block E  MBXHSF=MSIxMBXD15 assigned to mailbox handshake protocol block F  MBXHSG=MSIxMBXD15 assigned to mailbox handshake protocol block G  MBXHSH=MSIxMBXD15 assigned to mailbox handshake protocol block H  HSAEN=Mailbox data flow control handshake protocol block disabled  HSBEN=Mailbox data flow control handshake protocol block disabled  HSCEN=Mailbox data flow control handshake protocol block disabled  HSDEN=Mailbox data flow control handshake protocol block disabled  HSEEN=Mailbox data flow control handshake protocol block disabled  HSFEN=Mailbox data flow control handshake protocol block disabled  HSGEN=Mailbox data flow control handshake protocol block disabled  HSHEN=Mailbox data flow control handshake protocol block disabled  CPRA0=Master core owns pin  CPRA1=Master core owns pin  CPRA2=Master core owns pin  CPRA3=Master core owns pin  CPRA4=Master core owns pin  CPRB0=Master core owns pin  CPRB1=Master core owns pin  CPRB2=Master core owns pin  CPRB3=Master core owns pin  CPRB4=Master core owns pin  CPRB5=Master core owns pin  CPRB6=Master core owns pin  CPRB7=Master core owns pin  CPRB8=Master core owns pin  CPRB9=Master core owns pin  CPRB10=Master core owns pin  CPRB11=Master core owns pin  CPRB12=Master core owns pin  CPRB13=Master core owns pin  CPRB14=Master core owns pin  CPRB15=Master core owns pin  CPRC0=Master core owns pin  CPRC1=Master core owns pin  CPRC2=Master core owns pin  CPRC3=Master core owns pin  CPRC4=Master core owns pin  CPRC5=Master core owns pin  CPRC6=Master core owns pin  CPRC7=Master core owns pin  CPRC8=Master core owns pin  CPRC9=Master core owns pin  CPRC10=Master core owns pin  CPRC11=Master core owns pin  CPRC12=Master core owns pin  CPRC13=Master core owns pin  CPRC14=Master core owns pin  CPRC15=Master core owns pin  CPRD0=Master core owns pin  CPRD1=Master core owns pin  CPRD2=Master core owns pin  CPRD3=Master core owns pin  CPRD4=Master core owns pin  CPRD5=Master core owns pin  CPRD6=Master core owns pin  CPRD7=Master core owns pin  CPRD8=Master core owns pin  CPRD9=Master core owns pin  CPRD10=Master core owns pin  CPRD11=Master core owns pin  CPRD12=Master core owns pin  CPRD13=Master core owns pin  CPRD14=Master core owns pin  CPRD15=Master core owns pin  CPRE0=Master core owns pin  CPRE1=Master core owns pin  CPRE2=Master core owns pin  CPRE3=Master core owns pin  CPRE4=Master core owns pin  CPRE5=Master core owns pin  CPRE6=Master core owns pin  CPRE7=Master core owns pin  CPRE8=Master core owns pin  CPRE9=Master core owns pin  CPRE10=Master core owns pin  CPRE11=Master core owns pin  CPRE12=Master core owns pin  CPRE13=Master core owns pin  CPRE14=Master core owns pin  CPRE15=Master core owns pin  S1FNOSC=Internal Fast RC (FRC) Oscillator with postscaler  S1IESO=Start up with FRC; then switch  S1OSCIOFNC=OSC2 is clock output  S1FCKSM=Both Clock switching and Fail-safe Clock Monitor are disabled  S1PLLKEN=S1PLLKEN_ON  S1RWDTPS=1:1048576  S1RCLKSEL=Always use LPRC  S1WINDIS=Watchdog Timer operates in Non-Window mode  S1WDTWIN=WDT Window is 25% of WDT period  S1SWDTPS=1:1048576  S1FWDTEN=use WDTCON.ON bit  S1ICS=Communicate on PGC1 and PGD1  S1DEBUG=Not used  S1ISOLAT=The slave can operate (in debug mode) even if the SLVEN bit in the MSI is zero  S1NOBTSWP=BOOTSWP instruction is disabled  S1ALTI2C1=I2C1 mapped to SDA1/SCL1 pins  S1SPI1PIN=Slave SPI1 uses I/O remap (PPS) pins  S1SSRE=Slave generated resets will reset the Slave Enable Bit in the MSI module  S1MSRE=The master software oriented RESET events (RESET Op-Code; Watchdog timeout; TRAP reset; illegalInstruction) will also cause the slave subsystem to reset  S1CTXT1=Not Assigned  S1CTXT2=Not Assigned  S1CTXT3=Not Assigned  S1CTXT4=Not Assigned  BORLVL=Not used  BSSO=Not used  MCA=Not used  MAXTEMP=Not used  CFGAN14=Not used  CFGAN15=Not used  S1IOL1WAY=Not used  S1BSSO=Not used  S1BACKBUG=Not used  BISTDIS=mBIST on reset feature disabled  NOBTSWP=BOOTSWP instruction is disabled  S1BISTDIS=Slave BIST on reset feature disabled  S1DMTIVTL=Not used  S1DMTIVTH=Not used  S1DMTCNTL=Not used  S1DMTCNTH=Not used  S1DMTDIS=Slave Dead Man Timer is Disabled and can be enabled by software  BSEQ=Not used  IBSEQ=Not used  SMB3EN=SMBus 3.0 input levels  FUSBIDIO2=USBID pin is controlled by the USB2 module  FVBUSIO2=VBUSON pin is controlled by the USB2 module  FUSBIDIO1=USBID pin is controlled by the USB1 module  FVBUSIO1=VBUSON pin is controlled by the USB1 module  VBATBOREN=Enable ZPBOR during VBAT Mode  FDSEN=Enable DSEN bit in DSCON  BORSEL=BOR trip voltage 2.1v (Non-OPAMP deviced operation)  POSCFGAIN=Gain is G3  POSCAGCDLY=Settling time = 25ms x AGCRNG  POSCAGCRNG=Range 1x  POSCAGC=Automatic Gain Control for Oscillator  FDBGWP=Not used
      settings: SourceProductName=MPLAB® Device Blocks for Simulink®
  Open board Documentation : Subsystem
      settings: OpenFcn=|
      | web('http://www.microchip.com/DevelopmentTools/ProductDetails.aspx?PartNO=DM240001-2#utm_source=MicroSolutions&utm_medium=Link&utm_term=FY17Q3&utm_content=DevTools&utm_campaign=Article','-browser');
      | pause(1);
      | web('http://www.microchip.com/DevelopmentTools/ProductDetails.aspx?PartNO=MA330025-1','-browser');
      | pause(1);
      | web('http://microchipdeveloper.com/boards:explorer1632','-browser');
      | pause(1);
      | web('http://www.microchip.com/DevelopmentTools/ProductDetails.aspx?PartNO=MA330011','-browser');
      | pause(1);
      | web('http://ww1.microchip.com/downloads/en/DeviceDoc/Explorer_16_32_Schematics_R6_3.pdf','-browser');
      | pause(1);
      | web('http://microchipdeveloper.com/boards:explorer1632','-browser');
      | pause(1);
      | web('https://microchip.box.com/shared/static/0ohr115y3h27gpw3qhbe61d2urrmq4mz.pdf','-browser');
      mask Display: disp('Explorer 16/32\nDev Board');
  Port Info : MCHP_Blockset/System Info/Port Info  MCHP_MASTERLINK=Explorer1632_dsPIC33EP512MU810_UART_Terminal_R2017b/Explorer16//32 - dsPIC33EP512MU810/Microchip Master
      settings: SourceProductName=MPLAB® Device Blocks for Simulink®
  Simulink Reset Config : MCHP_Blockset/System Configuration/Simulink Reset Config  MCHP_MASTERLINK=0
      settings: SourceProductName=MPLAB® Device Blocks for Simulink®
  Timer Info : MCHP_Blockset/System Info/Timer Info  MCHP_MASTERLINK=Explorer1632_dsPIC33EP512MU810_UART_Terminal_R2017b/Explorer16//32 - dsPIC33EP512MU810/Microchip Master
      settings: SourceProductName=MPLAB® Device Blocks for Simulink®
  UART Configuration : MCHP_Blockset/BUS UART/UART Configuration  UART_REF=1  BAUD_Choice=Dynamic Options  BAUD_Choice_TXT="115200         [-0.06%]"  BAUD_Choice_IR=Dynamic Options  BAUD_Choice_IR_TXT=[]  BAUD_Custom=115200  INT_PRIORITY=0  ALT_IO=on  PIN_RX=Dynamic Options  PIN_RX_TXT=F4 / P100 / Pin[49]  PIN_TX=Dynamic Options  PIN_TX_TXT=F5 / P101 / Pin[50]  MCHP_PORT="{UART1  Rx}{U1RX}3:0:P100;{UART1  Tx}{U1TX}3:1:P101;"  MCHP_MASTERLINK=Explorer1632_dsPIC33EP512MU810_UART_Terminal_R2017b/Explorer16//32 - dsPIC33EP512MU810/Microchip Master  MCHP_COM_ExtPil=off  TX_IMPLEMENTATION=Circular Buffer  TX_IMPLEMENTATION_default=Circular Buffer  TX_INT_PRIORITY=6  TX_INT_WHEN=is empty  TX_INT_WHEN_default=is empty & last char is sent  TX_CIRCULAR_SIZE=2048  TX_DMA_CHANNEL="0   (Lowest Priority)"  TX_DMA_SIZE=[]  TX_TASK_PROTECTION=Delay tasks (default)  TX_INTERRUPT_PROTECTION=Do not send on conflict (default)  TX_INTERRUPT_PROTECTION_default=Do not send on conflict (default)  RX_IMPLEMENTATION=Simplest (4 bytes internal buffer only)  RX_IMPLEMENTATION_default=Circular Buffer  RX_INT_PRIORITY=5  RX_INT_WHEN=receive 1 character  RX_CIRCULAR_SIZE=128  RX_DMA_CHANNEL=0  RX_DMA_SIZE=0  DuplexMode=Full duplex (default)  PIN_RX_Inv=off  PIN_TX_Inv=off  PIN_RXTX_Inv=off  ParityBit=No parity (default)  StopBit=1 stop bit (default)  IRDA=off  FlowControl=None  PIN_CTS=Dynamic Options  PIN_CTS_TXT=A0 / P16 / Pin[17]  PIN_RTS=Dynamic Options  PIN_RTS_TXT=D0 / P64 / Pin[72]  InitSequence_chkbox=off  BAUD_Choice_InitSeq=Dynamic Options  BAUD_Choice_InitSeq_TXT="115200         [-0.06%]"  BAUD_Choice_IR_InitSeq=Dynamic Options  BAUD_Choice_IR_InitSeq_TXT=0  BAUD_Custom_InitSeq=0  InitSequence='Hello World'
      settings: SourceProductName=MPLAB® Device Blocks for Simulink®

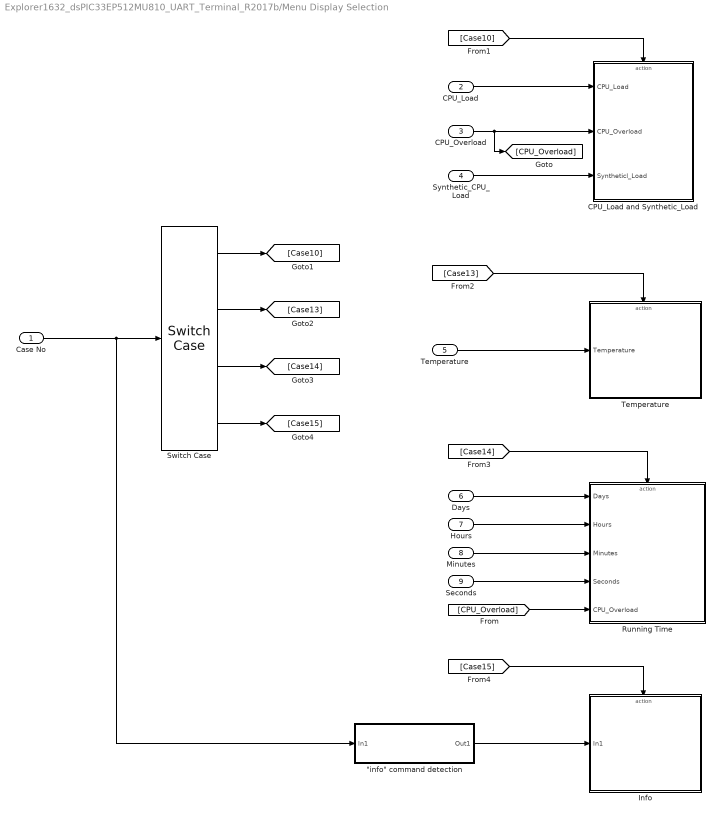
== system Explorer1632_dsPIC33EP512MU810_UART_Terminal_R2017b/Menu Display Selection ==
  Case No : Inport
  CPU_Load : Inport  Port=2
  CPU_Overload : Inport  Port=3
  Synthetic_CPU_Load : Inport  Port=4
  "Temperature " : Inport  Port=5
  Days : Inport  Port=6
  Hours : Inport  Port=7
  Minutes : Inport  Port=8
  Seconds : Inport  Port=9
  "\"info\" command detection" : Subsystem
  CPU_Load and Synthetic_Load : Subsystem  TreatAsAtomicUnit=on
  Info : Subsystem  TreatAsAtomicUnit=on
  Running Time : Subsystem  TreatAsAtomicUnit=on
  Switch Case : SwitchCase  CaseConditions={10,13,14,15}  ShowDefaultCase=off
  Temperature : Subsystem  TreatAsAtomicUnit=on
  wires:
  [Case10] -> CPU_Load and Synthetic_Load/Action
  CPU_Load/1 -> CPU_Load and Synthetic_Load/1(CPU_Load)
  Switch Case/1 -> [Case10]
  Switch Case/2 -> [Case13]
  "Temperature "/1 -> Temperature/1(Temperature)
  [Case13] -> Temperature/Action
  [Case14] -> Running Time/Action
  Switch Case/3 -> [Case14]
  Minutes/1 -> Running Time/3(Minutes)
  Hours/1 -> Running Time/2(Hours)
  Seconds/1 -> Running Time/4(Seconds)
  Days/1 -> Running Time/1(Days)
  Switch Case/4 -> [Case15]
  [Case15] -> Info/Action
  CPU_Overload/1 -> [CPU_Overload], CPU_Load and Synthetic_Load/2(CPU_Overload)
  Synthetic_CPU_Load/1 -> CPU_Load and Synthetic_Load/3(Syntheticl_Load)
  Case No/1 -> "\"info\" command detection"/1(In1), Switch Case/1
  "\"info\" command detection"/1(Out1) -> Info/1(In1)
  [CPU_Overload] -> Running Time/5(CPU_Overload)

== system Explorer1632_dsPIC33EP512MU810_UART_Terminal_R2017b/Snake LED D4-D10 ==
  "Counter Limited " : simulink/Sources/Counter Limited  uplimit=11  tsamp=.08
  Digital Output2 : MCHP_Blockset/Digital IO/Digital Output  PORT=Dynamic Options  PORT_TXT="A   [ 0  1  2  3  4  5  6  7  9  10  14  15 ]"  PIN=[1:7]  PACK=on  SIMULTANEOUS=off  READPREVIOUS=off  ORDERING=None  SampleTime=-1  MCHP_MASTERLINK=Explorer1632_dsPIC33EP512MU810_UART_Terminal_R2017b/Explorer16//32 - dsPIC33EP512MU810/Microchip Master
      settings: SourceProductName=MPLAB® Device Blocks for Simulink®
  Direct Lookup Table (n-D) : LookupNDDirect  NumberOfTableDimensions=1  Table=[ 2 4 8 16 32 64 128 64 32 16 8 4 ]  TableDataTypeStr=uint16
  wires:
  "Counter Limited "/1 -> Direct Lookup Table (n-D)/1
  Direct Lookup Table (n-D)/1 -> Digital Output2/1
